simulink model "SLXTest"  (R2024b)
settings: Solver=FixedStepAuto  StartTime=0.0  StopTime=inf  FixedStep=0.001  MaxStep=0.01  RelTol=1e-3  EnableMultiTasking=on
libraries: stm32f4xxblockslib x6, dspstat3 x4
settings Model: STM32="{\"AnalogInput\":[{\"ID\":\"SLXTest:1\"},{\"ID\":\"SLXTest:27\"},{\"ID\":\"SLXTest:29\"}],\"DigitalPortRead\":[{\"ID\":\"SLXTest:14\"},{\"ID\":\"SLXTest:45\"}],\"DigitalPortWrite\":{\"ID\":\"SLXTest:15\"}}"  Creator=KATANA  LastModifiedBy=KATANA
settings SolverCC: AllowMultiTaskInputOutput=on
settings OptimizationCC: EnhancedBackFolding=on  PassReuseOutputArgsAs=Individual arguments  ZeroExternalMemoryAtStartup=off  ZeroInternalMemoryAtStartup=off  MaxStackSize=512  OptimizeBlockOrder=speed  DifferentSizesBufferReuse=on  OptimizationCustomize=off  EfficientTunableParamExpr=on
settings DebuggingCC: ParameterTunabilityLossMsg=error
settings HardwareCC: ProdBitPerPointer=32  ProdBitPerSizeT=32  ProdBitPerPtrDiffT=32  ProdLargestAtomicInteger=Long  ProdLargestAtomicFloat=Double  ProdWordSize=32  ProdLongLongMode=on  ProdHWDeviceType=ARM Compatible->ARM Cortex-M
settings SFSimCC: MATLABDynamicMemAlloc=off
settings RTWCC: Description=Embedded Coder  SystemTargetFile=ert.tlc  HardwareBoard=STM32G4xx Based  TemplateMakefile=ert_default_tmf  Toolchain=GNU Tools for ARM Embedded Processors
settings CodeAppCC: ForceParamTrailComments=on  IgnoreCustomStorageClasses=off  OperatorAnnotations=on  SimulinkDataObjDesc=on  SFDataObjDesc=on  InsertBlockDesc=on
settings ERTTargetCC: TargetLangStandard=C99 (ISO)  CodeReplacementLibrary=ARM Cortex-M  ExtModeTransport=3  ExtModeStaticAlloc=on  ExtModeStaticAllocSize=2048  ExtModeMexFile=ext_xcp  ExtModeIntrfLevel=Level2 - Open  InlinedParameterPlacement=Hierarchical  DynamicArrayContainerType=coder::array

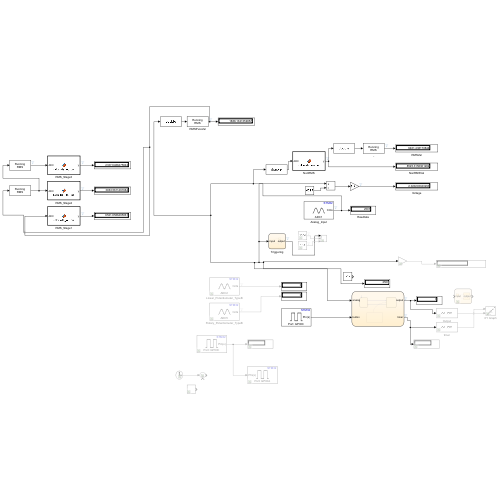
[thumbnail: Simulink's stored preview of the top-level diagram]
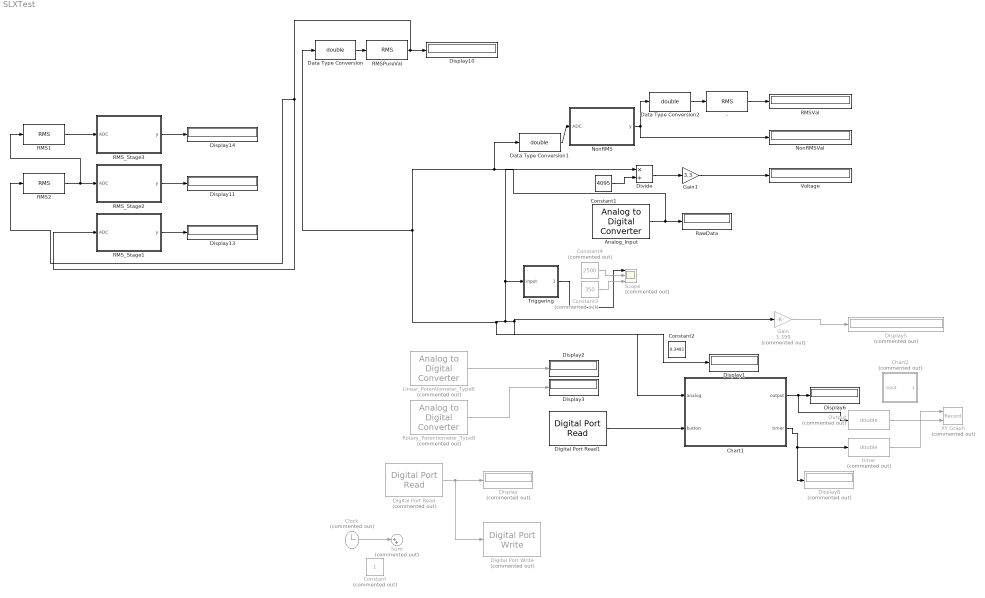
== system SLXTest ==
  - : dspstat3/RMS  run=on  directionMode=Entire input  dimension=1  reset_popup=None
  Analog_Input : stm32f4xxblockslib/Analog to Digital Converter  ADCModule=ADC1  ConversionGroup=Regular  TriggerMode=Trigger and read  NumberOfConversions=1  EnableBufferConv=off  BufferLength=1  OutputStatus=off  SampleTime=-1  EnableSimPort=off  hoistedMaskSrc=ECSoC/ECSimCodegen/Analog to Digital Converter
  Chart1 : Stateflow chart  TreatAsAtomicUnit=on
  Chart2 : Stateflow chart  Commented=on  TreatAsAtomicUnit=on
  Clock : Clock  Commented=on
  Constant : Constant  Commented=on
  Constant1 : Constant  Value=4095
  Constant2 : Constant  Value=0.3481
  Constant3 : Constant  Commented=on  Value=350
  Constant4 : Constant  Commented=on  Value=2500
  Data Type Conversion : DataTypeConversion  OutDataTypeStr=double  SaturateOnIntegerOverflow=off  RndMeth=Floor
  Data Type Conversion1 : DataTypeConversion  OutDataTypeStr=double  SaturateOnIntegerOverflow=off  RndMeth=Floor
  Data Type Conversion2 : DataTypeConversion  OutDataTypeStr=double  SaturateOnIntegerOverflow=off  RndMeth=Floor
  Digital Port Read : stm32f4xxblockslib/Digital Port Read  Commented=on  PortName=GPIOC  PinNumber=[13]  ReadOperation=on  IOAsArray=on  SampleTime=-1  EnableSimPort=off  hoistedMaskSrc=ECSoC/ECSimCodegen/Digital Port Read
      settings: LibrarySourceBlock=stm32g4xxblockslib/Digital Port Read
  Digital Port Read1 : stm32f4xxblockslib/Digital Port Read  PortName=GPIOC  PinNumber=13  ReadOperation=on  IOAsArray=on  SampleTime=-1  EnableSimPort=off  hoistedMaskSrc=ECSoC/ECSimCodegen/Digital Port Read
      settings: LibrarySourceBlock=stm32g4xxblockslib/Digital Port Read
  Digital Port Write : stm32f4xxblockslib/Digital Port Write  Commented=on  PortName=GPIOA  PinNumber=[5]  ReadOperation=off  IOAsArray=on  EnableSimPort=off  hoistedMaskSrc=ECSoC/ECSimCodegen/Digital Port Write
      settings: LibrarySourceBlock=stm32g4xxblockslib/Digital Port Write
  Display : Display  Commented=on
  Display{1..3,6,10..11,13..14} (8 alike) : Display
  Display5 : Display  Commented=on
      settings: Decimation=2
  Display8 : Display  Commented=on
  Divide : Product  Inputs=*/
  Gain : Gain  Commented=on  Gain=3.399
  Gain1 : Gain  Gain=3.3
  Linear_Potentiometer_TypeB : stm32f4xxblockslib/Analog to Digital Converter  Commented=on  ADCModule=ADC2  ConversionGroup=Regular  TriggerMode=Trigger and read  NumberOfConversions=1  EnableBufferConv=off  BufferLength=1  OutputStatus=off  SampleTime=-1  EnableSimPort=off  hoistedMaskSrc=ECSoC/ECSimCodegen/Analog to Digital Converter
  NonRMS : MATLAB Function  TreatAsAtomicUnit=on
  NonRMSVal : Display
  Output : DataTypeConversion  Commented=on  OutDataTypeStr=double  SaturateOnIntegerOverflow=off  RndMeth=Floor
  RMS1 : dspstat3/RMS  run=on  directionMode=Entire input  dimension=1  reset_popup=None
  RMS2 : dspstat3/RMS  run=on  directionMode=Entire input  dimension=1  reset_popup=None
  RMSPureVal : dspstat3/RMS  run=on  directionMode=Entire input  dimension=1  reset_popup=None
  RMSVal : Display
  RMS_Stage1 : MATLAB Function  TreatAsAtomicUnit=on
  RMS_Stage2 : MATLAB Function  TreatAsAtomicUnit=on
  RMS_Stage3 : MATLAB Function  TreatAsAtomicUnit=on
  RawData : Display
  Rotary_Potentiometer_TypeB : stm32f4xxblockslib/Analog to Digital Converter  Commented=on  ADCModule=ADC5  ConversionGroup=Regular  TriggerMode=Trigger and read  NumberOfConversions=1  EnableBufferConv=off  BufferLength=1  OutputStatus=off  SampleTime=-1  EnableSimPort=off  hoistedMaskSrc=ECSoC/ECSimCodegen/Analog to Digital Converter
  Scope : Scope  Commented=on  NumInputPorts=3
  Sum : Sum  Commented=on  Inputs=|++
  Triggering : Stateflow chart  TreatAsAtomicUnit=on
  Voltage : Display
  XY Graph : Record  Commented=on  FileSettingsInternal="{\"entries\":[{\"content\":{\"excelSettings\":{\"content\":{},\"type\":\"Streamout.ExcelSettings\"}},\"type\":\"Streamout.FileSettingStorage\",\"uuid\":\"\"}],\"packageUris\":[\"http:\\/\\/schema.mathworks.com\\/mf0\\/streamout_blocks\\/R2020a\"],\"version\":\"1.0\"}"  Layout=[1 1]  SignalsInternal="{\"entries\":[{\"content\":{},\"type\":\"RecordBlkView.InputSignals\",\"uuid\":\"\"}],\"packageUris\":[\"http:\\/\\/schema.mathworks.com\\/mf0\\/streamout_blocks\\/R2020a\"],\"version\":\"1.0\"}"  VisualizationBindings="{\"xyplotplugin\":{\"info\":[{\"series\":[],\"subplotID\":1}]}}"  CompatibilityTag=XY
  timer : DataTypeConversion  Commented=on  OutDataTypeStr=double  SaturateOnIntegerOverflow=off  RndMeth=Floor
  wires:
  Clock/1 -> Sum/1
  Digital Port Read/1 -> Digital Port Write/1, Display/1
  Linear_Potentiometer_TypeB/1 -> Display2/1
  Rotary_Potentiometer_TypeB/1 -> Display3/1
  Triggering/1(output) -> Scope/1
  Gain/1 -> Display5/1
  Analog_Input/1 -> RawData/1, Chart1/1(analog), Divide/1, Data Type Conversion1/1, Data Type Conversion/1, Display1/1, Gain/1, Triggering/1(input)
  Digital Port Read1/1 -> Chart1/2(button)
  Constant1/1 -> Divide/2
  Divide/1 -> Gain1/1
  Gain1/1 -> Voltage/1
  Chart1/1(output) -> Output/1, Display6/1
  Chart1/2(timer) -> Display8/1, timer/1
  Output/1 -> XY Graph/2
  timer/1 -> XY Graph/1
  RMSPureVal/1 -> RMS_Stage1/1(ADC), RMS2/1, Display10/1
  Data Type Conversion/1 -> RMSPureVal/1
  NonRMS/1(y) -> NonRMSVal/1, Data Type Conversion2/1
  Data Type Conversion1/1 -> NonRMS/1(ADC)
  -/1 -> RMSVal/1
  Data Type Conversion2/1 -> -/1
  RMS_Stage1/1(y) -> Display13/1
  RMS2/1 -> RMS1/1, RMS_Stage2/1(ADC)
  RMS1/1 -> RMS_Stage3/1(ADC)
  RMS_Stage2/1(y) -> Display11/1
  RMS_Stage3/1(y) -> Display14/1
  Constant3/1 -> Scope/3
  Constant4/1 -> Scope/2

== stateflow chart SLXTest/Chart1 ==
  state Do
    during:
    timer = timer + 0.01;
    output = analog
    time = time + 0.01;
  state Initial
    entry:
    timer = 0;
    during:
    time = 0;
    output = 0;
  state Idle1 [commented out]
    time = 0;
    output = 0;
  (default) -> Initial
  Initial -> Do : [button == 1]
  Idle1 -> Do [commented out] : [button == 1]
  Do -> Initial : [time >= 0.99]
  data: analog input; button input; output output uint16; time local; timer output

== stateflow chart SLXTest/Chart2 ==
  state Case1
    ouput =
  state Initial
    input;
    output;
  state Case2
    output = (input +126.47)/0.3089;
  (default) -> Initial
  Initial -> Case1 [order 1] : [input <= 328.5456]
  Initial -> Case2 [order 2] : [input > 328.5456]
  Case2 -> Case1 : [input <= 328.5456]
  Case1 -> Case2 : [input > 328.5456]
  data: input input; output output

== stateflow chart SLXTest/Triggering ==
  state Nontrig
    %entry:
    %time = 0;
    output = 0;
    %during:
    %time = time + 0.01
  state Initial
    input;
    %time = 0;
    output = 0;
  state Trig
    output = 4095;
    %entry:
    %time = 0;
    %during:
    %time = time + 0.01
  Initial -> Nontrig [order 1] : [input <= 350]
  (default) -> Initial
  Nontrig -> Trig : [[input >2500]]
  Trig -> Nontrig : [[ input <= 350]]
  Initial -> Trig [order 2] : [input >2500]
  data: output output; input input

== matlab function SLXTest/NonRMS ==
  data: ADC input; y output
function y = calculate_output(ADC)
% Input:
% ADC - ค่า ADC ที่รับเข้ามา
% Output:
% y - ค่าที่คำนวณได้ตามเงื่อนไขของ ADC

    if ADC < 328
        % ตั้งค่าคงที่ในสมการพหุนาม
        coefficients = [-2e-17, 6e-14, -8e-11, 3e-8, 0.0002, 0.0158, 2.6752];
        y_target = ADC; % กำหนด y เป็นค่า ADC

        % ฟังก์ชันที่ใช้ในการหาค่า x ที่ทำให้ y ใกล้เคียงกับ ADC
        polynomial_func = @(x) polyval(coefficients, x) - y_target;

        % หา x โดยใช้ fzero โดยให้ค่าเริ่มต้น
        x_guess = 0;
        x = fzero(polynomial_func, x_guess);
        
        % คืนค่า y เป็นค่า x ที่คำนวณได้
        y = x; % คืนค่าที่ได้จาก x
        if y < 0
            y = 0; % ถ้า y น้อยกว่า 0 ให้คืนค่าเป็น 0
        end
    else
        % ถ้า ADC มากกว่า 328 ใช้สมการเชิงเส้นเพื่อคำนวณ y
        y = (ADC + 126.47) / 0.3089; % คำนวณ x
    end
end

== matlab function SLXTest/RMS_Stage1 ==
  data: ADC input; y output
function y = calculate_output(ADC)
% Input:
% ADC - ค่า ADC ที่รับเข้ามา
% Output:
% y - ค่าที่คำนวณได้ตามเงื่อนไขของ ADC

    if ADC < 328
        % ตั้งค่าคงที่ในสมการพหุนาม
        coefficients = [-2e-17, 6e-14, -8e-11, 3e-8, 0.0002, 0.0158, 2.6752];
        y_target = ADC; % กำหนด y เป็นค่า ADC

        % ฟังก์ชันที่ใช้ในการหาค่า x ที่ทำให้ y ใกล้เคียงกับ ADC
        polynomial_func = @(x) polyval(coefficients, x) - y_target;

        % หา x โดยใช้ fzero โดยให้ค่าเริ่มต้น
        x_guess = 0;
        x = fzero(polynomial_func, x_guess);
        
        % คืนค่า y เป็นค่า x ที่คำนวณได้
        y = x; % คืนค่าที่ได้จาก x
        if y < 0
            y = 0; % ถ้า y น้อยกว่า 0 ให้คืนค่าเป็น 0
        end
    else
        % ถ้า ADC มากกว่า 328 ใช้สมการเชิงเส้นเพื่อคำนวณ y
        y = (ADC + 126.47) / 0.3089; % คำนวณ x
    end
end

== matlab function SLXTest/RMS_Stage2 ==
  data: ADC input; y output
function y = calculate_output(ADC)
% Input:
% ADC - ค่า ADC ที่รับเข้ามา
% Output:
% y - ค่าที่คำนวณได้ตามเงื่อนไขของ ADC

    if ADC < 328
        % ตั้งค่าคงที่ในสมการพหุนาม
        coefficients = [-2e-17, 6e-14, -8e-11, 3e-8, 0.0002, 0.0158, 2.6752];
        y_target = ADC; % กำหนด y เป็นค่า ADC

        % ฟังก์ชันที่ใช้ในการหาค่า x ที่ทำให้ y ใกล้เคียงกับ ADC
        polynomial_func = @(x) polyval(coefficients, x) - y_target;

        % หา x โดยใช้ fzero โดยให้ค่าเริ่มต้น
        x_guess = 0;
        x = fzero(polynomial_func, x_guess);
        
        % คืนค่า y เป็นค่า x ที่คำนวณได้
        y = x; % คืนค่าที่ได้จาก x
        if y < 0
            y = 0; % ถ้า y น้อยกว่า 0 ให้คืนค่าเป็น 0
        end
    else
        % ถ้า ADC มากกว่า 328 ใช้สมการเชิงเส้นเพื่อคำนวณ y
        y = (ADC + 126.47) / 0.3089; % คำนวณ x
    end
end

== matlab function SLXTest/RMS_Stage3 ==
  data: ADC input; y output
function y = calculate_output(ADC)
% Input:
% ADC - ค่า ADC ที่รับเข้ามา
% Output:
% y - ค่าที่คำนวณได้ตามเงื่อนไขของ ADC

    if ADC < 328
        % ตั้งค่าคงที่ในสมการพหุนาม
        coefficients = [-2e-17, 6e-14, -8e-11, 3e-8, 0.0002, 0.0158, 2.6752];
        y_target = ADC; % กำหนด y เป็นค่า ADC

        % ฟังก์ชันที่ใช้ในการหาค่า x ที่ทำให้ y ใกล้เคียงกับ ADC
        polynomial_func = @(x) polyval(coefficients, x) - y_target;

        % หา x โดยใช้ fzero โดยให้ค่าเริ่มต้น
        x_guess = 0;
        x = fzero(polynomial_func, x_guess);
        
        % คืนค่า y เป็นค่า x ที่คำนวณได้
        y = x; % คืนค่าที่ได้จาก x
        if y < 0
            y = 0; % ถ้า y น้อยกว่า 0 ให้คืนค่าเป็น 0
        end
    else
        % ถ้า ADC มากกว่า 328 ใช้สมการเชิงเส้นเพื่อคำนวณ y
        y = (ADC + 126.47) / 0.3089; % คำนวณ x
    end
end
